simulink model "IEEE30_case"  (R2024b)
settings: Solver=FixedStepAuto  StartTime=0  StopTime=5  FixedStep=1e-7  RelTol=1e-3
values from neighbouring files (symbols this model uses):
  GFL_DFIG_7_C_bus = 0.08    [IEEE30_case_parameters.m]
  GFL_DFIG_7_D_mutual = 2.500000e+3    (= 2500)    [IEEE30_case_parameters.m]
  GFL_DFIG_7_f0 = 60    [IEEE30_case_parameters.m]
  GFL_DFIG_7_gPLLi = 3200    [IEEE30_case_parameters.m]
  GFL_DFIG_7_gPLLp = 650    [IEEE30_case_parameters.m]
  GFL_DFIG_7_H_WT = 0.4    [IEEE30_case_parameters.m]
  GFL_DFIG_7_Hg = 0.8    [IEEE30_case_parameters.m]
  GFL_DFIG_7_Igq_ref = 0    [IEEE30_case_parameters.m]
  GFL_DFIG_7_Ird_ref = 704.45696    [IEEE30_case_parameters.m]
  GFL_DFIG_7_KI_V = -300000    [IEEE30_case_parameters.m]
  GFL_DFIG_7_KP_V = -1000    [IEEE30_case_parameters.m]
  GFL_DFIG_7_Ksh = 1.254300e+4    (= 12543)    [IEEE30_case_parameters.m]
  GFL_DFIG_7_Lg = 0.000483    [IEEE30_case_parameters.m]
  GFL_DFIG_7_Lm_pu = 4    [IEEE30_case_parameters.m]
  GFL_DFIG_7_N = 100    [IEEE30_case_parameters.m]
  GFL_DFIG_7_p = 2    [IEEE30_case_parameters.m]
  GFL_DFIG_7_Pitch = 0    [IEEE30_case_parameters.m]
  GFL_DFIG_7_R = 44    [IEEE30_case_parameters.m]
  GFL_DFIG_7_Rg = 2.000000e-5    (= 2e-05)    [IEEE30_case_parameters.m]
  GFL_DFIG_7_rho = 1.225    [IEEE30_case_parameters.m]
  GFL_DFIG_7_rPLLi = 4500    [IEEE30_case_parameters.m]
  GFL_DFIG_7_rPLLp = 620    [IEEE30_case_parameters.m]
  GFL_DFIG_7_Rs_pu = 0.011    [IEEE30_case_parameters.m]
  GFL_DFIG_7_Sbase = 2.000000e+6    (= 2000000)    [IEEE30_case_parameters.m]
  GFL_DFIG_7_ugq_ref = 0    [IEEE30_case_parameters.m]
  GFL_DFIG_7_usd_ref = 0    [IEEE30_case_parameters.m]
  GFL_DFIG_7_Vbase = 690    [IEEE30_case_parameters.m]
  GFL_DFIG_7_Vdc_ref = 1200    [IEEE30_case_parameters.m]
  GFL_DFIG_7_wind = 12    [IEEE30_case_parameters.m]
  GFL_DFIG_7_wm_ref = 518.184209    [IEEE30_case_parameters.m]
  SG_D_13_D = 0.01056    [IEEE30_case_parameters.m]
  SG_D_13_EnableSaturation = 0    [IEEE30_case_parameters.m]
  SG_D_13_f0 = 60    [IEEE30_case_parameters.m]
  SG_D_13_H = 7.5    [IEEE30_case_parameters.m]
  SG_D_13_K_A = 20    [IEEE30_case_parameters.m]
  SG_D_13_K_E = 1.000000e+1    (= 10)    [IEEE30_case_parameters.m]
  SG_D_13_K_F = 2.363    [IEEE30_case_parameters.m]
  SG_D_13_K_s = 0.5    [IEEE30_case_parameters.m]
  SG_D_13_R_a = 0.001088    [IEEE30_case_parameters.m]
  SG_D_13_S_A = 1    [IEEE30_case_parameters.m]
  SG_D_13_S_B = 0.103    [IEEE30_case_parameters.m]
  SG_D_13_S_N = 10.659857    [IEEE30_case_parameters.m]
  SG_D_13_SpeedPara = 200    [IEEE30_case_parameters.m]
  SG_D_13_T_0 = 0.370163    [IEEE30_case_parameters.m]
  SG_D_13_T_1 = 0.3    [IEEE30_case_parameters.m]
  SG_D_13_T_2 = 0.05    [IEEE30_case_parameters.m]
  SG_D_13_T_3 = 0.02    [IEEE30_case_parameters.m]
  SG_D_13_T_4 = 0.005    [IEEE30_case_parameters.m]
  SG_D_13_T_A = 0.02    [IEEE30_case_parameters.m]
  SG_D_13_T_dd = 8.000000e+0    (= 8)    [IEEE30_case_parameters.m]
  SG_D_13_T_ddd = 0.04    [IEEE30_case_parameters.m]
  SG_D_13_T_E = 0.314    [IEEE30_case_parameters.m]
  SG_D_13_T_F = 0.35    [IEEE30_case_parameters.m]
  SG_D_13_T_qd = 0.8    [IEEE30_case_parameters.m]
  SG_D_13_T_qdd = 0.02    [IEEE30_case_parameters.m]
  SG_D_13_T_speed = 0.1    [IEEE30_case_parameters.m]
  SG_D_13_T_w = 0.5    [IEEE30_case_parameters.m]
  SG_D_13_V_ref = 1.696619    [IEEE30_case_parameters.m]
  SG_D_13_w_ref = 376.991118    [IEEE30_case_parameters.m]
  SG_D_13_x_d = 1.9    [IEEE30_case_parameters.m]
  SG_D_13_x_dd = 0.302    [IEEE30_case_parameters.m]
  SG_D_13_x_ddd = 0.204    [IEEE30_case_parameters.m]
  SG_D_13_x_l = 0.05    [IEEE30_case_parameters.m]
  SG_D_13_x_q = 1.3    [IEEE30_case_parameters.m]
  SG_D_13_x_qd = 0.5    [IEEE30_case_parameters.m]
  SG_D_13_x_qdd = 0.3    [IEEE30_case_parameters.m]
  SG_D_1_D = 0.01056    [IEEE30_case_parameters.m]
  SG_D_1_EnableSaturation = 0    [IEEE30_case_parameters.m]
  SG_D_1_f0 = 60    [IEEE30_case_parameters.m]
  SG_D_1_H = 7.5    [IEEE30_case_parameters.m]
  SG_D_1_K_A = 20    [IEEE30_case_parameters.m]
  SG_D_1_K_E = 1.000000e+1    (= 10)    [IEEE30_case_parameters.m]
  SG_D_1_K_F = 2.363    [IEEE30_case_parameters.m]
  SG_D_1_K_s = 0.5    [IEEE30_case_parameters.m]
  SG_D_1_R_a = 0.001088    [IEEE30_case_parameters.m]
  SG_D_1_S_A = 1    [IEEE30_case_parameters.m]
  SG_D_1_S_B = 0.103    [IEEE30_case_parameters.m]
  SG_D_1_S_N = 10.659857    [IEEE30_case_parameters.m]
  SG_D_1_SpeedPara = 200    [IEEE30_case_parameters.m]
  SG_D_1_T_0 = 0.259812    [IEEE30_case_parameters.m]
  SG_D_1_T_1 = 0.3    [IEEE30_case_parameters.m]
  SG_D_1_T_2 = 0.05    [IEEE30_case_parameters.m]
  SG_D_1_T_3 = 0.02    [IEEE30_case_parameters.m]
  SG_D_1_T_4 = 0.005    [IEEE30_case_parameters.m]
  SG_D_1_T_A = 0.02    [IEEE30_case_parameters.m]
  SG_D_1_T_dd = 8.000000e+0    (= 8)    [IEEE30_case_parameters.m]
  SG_D_1_T_ddd = 0.04    [IEEE30_case_parameters.m]
  SG_D_1_T_E = 0.314    [IEEE30_case_parameters.m]
  SG_D_1_T_F = 0.35    [IEEE30_case_parameters.m]
  SG_D_1_T_qd = 0.8    [IEEE30_case_parameters.m]
  SG_D_1_T_qdd = 0.02    [IEEE30_case_parameters.m]
  SG_D_1_T_speed = 0.1    [IEEE30_case_parameters.m]
  SG_D_1_T_w = 0.5    [IEEE30_case_parameters.m]
  SG_D_1_V_ref = 1.544107    [IEEE30_case_parameters.m]
  SG_D_1_w_ref = 376.991118    [IEEE30_case_parameters.m]
  SG_D_1_x_d = 1.9    [IEEE30_case_parameters.m]
  SG_D_1_x_dd = 0.302    [IEEE30_case_parameters.m]
  SG_D_1_x_ddd = 0.204    [IEEE30_case_parameters.m]
  SG_D_1_x_l = 0.05    [IEEE30_case_parameters.m]
  SG_D_1_x_q = 1.3    [IEEE30_case_parameters.m]
  SG_D_1_x_qd = 0.5    [IEEE30_case_parameters.m]
  SG_D_1_x_qdd = 0.3    [IEEE30_case_parameters.m]
  SG_D_22_D = 0.01056    [IEEE30_case_parameters.m]
  SG_D_22_EnableSaturation = 0    [IEEE30_case_parameters.m]
  SG_D_22_f0 = 60    [IEEE30_case_parameters.m]
  SG_D_22_H = 7.5    [IEEE30_case_parameters.m]
  SG_D_22_K_A = 20    [IEEE30_case_parameters.m]
  SG_D_22_K_E = 1.000000e+1    (= 10)    [IEEE30_case_parameters.m]
  SG_D_22_K_F = 2.363    [IEEE30_case_parameters.m]
  SG_D_22_K_s = 0.5    [IEEE30_case_parameters.m]
  SG_D_22_R_a = 0.001088    [IEEE30_case_parameters.m]
  SG_D_22_S_A = 1    [IEEE30_case_parameters.m]
  SG_D_22_S_B = 0.103    [IEEE30_case_parameters.m]
  SG_D_22_S_N = 10.659857    [IEEE30_case_parameters.m]
  SG_D_22_SpeedPara = 200    [IEEE30_case_parameters.m]
  SG_D_22_T_0 = 0.216121    [IEEE30_case_parameters.m]
  SG_D_22_T_1 = 0.3    [IEEE30_case_parameters.m]
  SG_D_22_T_2 = 0.05    [IEEE30_case_parameters.m]
  SG_D_22_T_3 = 0.02    [IEEE30_case_parameters.m]
  SG_D_22_T_4 = 0.005    [IEEE30_case_parameters.m]
  ... (+126 more)
(part 14 of 27)

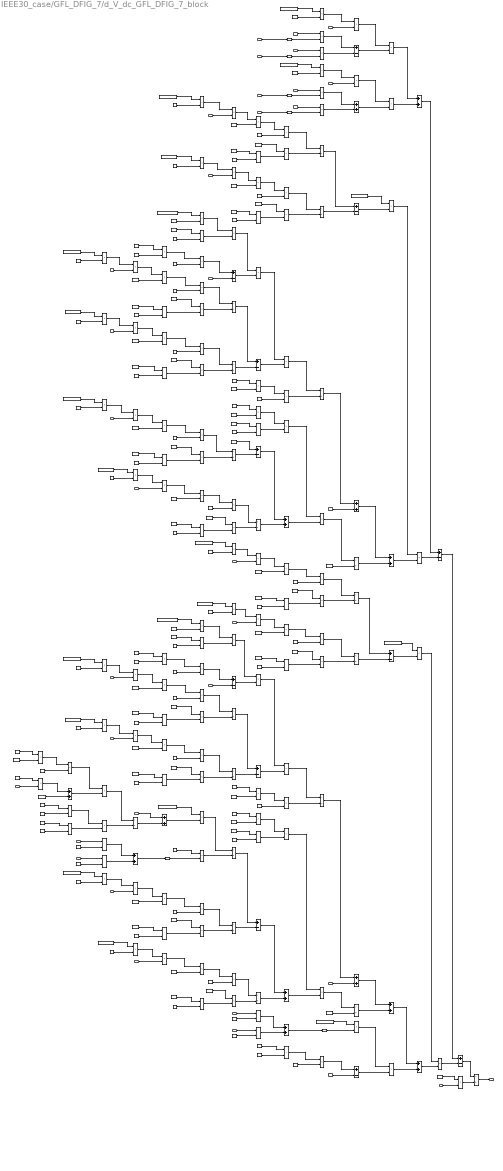
== system IEEE30_case/GFL_DFIG_7/d_V_dc_GFL_DFIG_7_block ==
  note: d_V_dc_GFL_DFIG_7 in IEEE30_case
      | $-\frac{\left(\frac{174.06679757657410473909892168\,\pi \,\Psi _{\mathrm{dr},\mathrm{GFL},\mathrm{DFIG},7}\,\mathrm{Sbase}\,f_{0}}{\mathrm{Lm}_{\mathrm{pu}}\,{\mathrm{Vbase}}^2}-\frac{172.34336393720189526090107832\,\pi \,\Psi _{\mathrm{ds},\mathrm{GFL},\mathrm{DFIG},7}\,\mathrm{Sbase}\,f_{0}}{\mathrm{Lm}_{\mathrm{pu}}\,{\mathrm{Vbase}}^2}\right)\,\left(\Phi _{\mathrm{ra},\mathrm{GFL},\mathrm{DFIG},7}+\frac{1.1\,\mathrm{Rs}_{\mathrm{pu}}\,{\mathrm{Vbase}}^2\,\left(\mathrm{Ird}_{\mathrm{ref}}-\frac{100.497512437811\,\pi \,\Psi _{\mathrm{dr},\mathrm{GFL},\mathrm{DFIG},7}\,\mathrm{Sbase}\,f_{0}}{\mathrm{Lm}_{\mathrm{pu}}\,{\mathrm{Vbase}}^2}+\frac{99.502487562189\,\pi \,\Psi _{\mathrm{ds},\mathrm{GFL},\mathrm{DFIG},7}\,\mathrm{Sbase}\,f_{0}}{\mathrm{Lm}_{\mathrm{pu}}\,{\mathrm{Vbase}}^2}\right)}{\mathrm{Sbase}}+\frac{0.00995049504950496\,\mathrm{Lm}_{\mathrm{pu}}\,{\mathrm{Vbase}}^2\,\left(\frac{100.497512437811\,\pi \,\Psi _{\mathrm{qr},\mathrm{GFL},\mathrm{DFIG},7}\,\mathrm{Sbase}\,f_{0}}{\mathrm{Lm}_{\mathrm{pu}}\,{\mathrm{Vbase}}^2}-\frac{99.502487562189\,\pi \,\Psi _{\mathrm{qs},\mathrm{GFL},\mathrm{DFIG},7}\,\mathrm{Sbase}\,f_{0}}{\mathrm{Lm}_{\mathrm{pu}}\,{\mathrm{Vbase}}^2}\right)\,\left(w_{m,\mathrm{GFL},\mathrm{DFIG},7}-2\,\pi \,f_{0}\right)}{\mathrm{Sbase}\,f_{0}\,\pi }\right)-\left(\frac{174.06679757657410473909892168\,\pi \,\Psi _{\mathrm{qr},\mathrm{GFL},\mathrm{DFIG},7}\,\mathrm{Sbase}\,f_{0}}{\mathrm{Lm}_{\mathrm{pu}}\,{\mathrm{Vbase}}^2}-\frac{172.34336393720189526090107832\,\pi \,\Psi _{\mathrm{qs},\mathrm{GFL},\mathrm{DFIG},7}\,\mathrm{Sbase}\,f_{0}}{\mathrm{Lm}_{\mathrm{pu}}\,{\mathrm{Vbase}}^2}\right)\,\left(0.99009900990099\,\sqrt{{\Psi _{\mathrm{ds},\mathrm{GFL},\mathrm{DFIG},7}}^2+{\Psi _{\mathrm{qs},\mathrm{GFL},\mathrm{DFIG},7}}^2}\,\left(w_{m,\mathrm{GFL},\mathrm{DFIG},7}-2\,\pi \,f_{0}\right)-\Phi _{\mathrm{rb},\mathrm{GFL},\mathrm{DFIG},7}+\frac{1.1\,\mathrm{Rs}_{\mathrm{pu}}\,{\mathrm{Vbase}}^2\,\left(\frac{0.673333333333333\,\Phi _{\mathrm{rc},\mathrm{GFL},\mathrm{DFIG},7}-\frac{10.773333333333328\,\mathrm{Sbase}\,p\,\left(w_{m,\mathrm{GFL},\mathrm{DFIG},7}-\mathrm{wm}_{\mathrm{ref}}\right)}{{f_{0}}^2\,\pi ^2}}{p\,\sqrt{{\Psi _{\mathrm{ds},\mathrm{GFL},\mathrm{DFIG},7}}^2+{\Psi _{\mathrm{qs},\mathrm{GFL},\mathrm{DFIG},7}}^2}}+\frac{100.497512437811\,\pi \,\Psi _{\mathrm{qr},\mathrm{GFL},\mathrm{DFIG},7}\,\mathrm{Sbase}\,f_{0}}{\mathrm{Lm}_{\mathrm{pu}}\,{\mathrm{Vbase}}^2}-\frac{99.502487562189\,\pi \,\Psi _{\mathrm{qs},\mathrm{GFL},\mathrm{DFIG},7}\,\mathrm{Sbase}\,f_{0}}{\mathrm{Lm}_{\mathrm{pu}}\,{\mathrm{Vbase}}^2}\right)}{\mathrm{Sbase}}+\frac{0.00995049504950496\,\mathrm{Lm}_{\mathrm{pu}}\,{\mathrm{Vbase}}^2\,\left(\frac{100.497512437811\,\pi \,\Psi _{\mathrm{dr},\mathrm{GFL},\mathrm{DFIG},7}\,\mathrm{Sbase}\,f_{0}}{\mathrm{Lm}_{\mathrm{pu}}\,{\mathrm{Vbase}}^2}-\frac{99.502487562189\,\pi \,\Psi _{\mathrm{ds},\mathrm{GFL},\mathrm{DFIG},7}\,\mathrm{Sbase}\,f_{0}}{\mathrm{Lm}_{\mathrm{pu}}\,{\mathrm{Vbase}}^2}\right)\,\left(w_{m,\mathrm{GFL},\mathrm{DFIG},7}-2\,\pi \,f_{0}\right)}{\mathrm{Sbase}\,f_{0}\,\pi }\right)+1.73205080756888\,\mathrm{Vbase}\,i_{\mathrm{gd},\mathrm{GFL},\mathrm{DFIG},7}\,\left(v_{d,\mathrm{GFL},\mathrm{DFIG},7}\,\cos\left(\theta _{\mathrm{pllg},\mathrm{GFL},\mathrm{DFIG},7}\right)-v_{q,\mathrm{GFL},\mathrm{DFIG},7}\,\sin\left(\theta _{\mathrm{pllg},\mathrm{GFL},\mathrm{DFIG},7}\right)\right)-1.73205080756888\,\mathrm{Vbase}\,i_{\mathrm{gq},\mathrm{GFL},\mathrm{DFIG},7}\,\left(v_{q,\mathrm{GFL},\mathrm{DFIG},7}\,\cos\left(\theta _{\mathrm{pllg},\mathrm{GFL},\mathrm{DFIG},7}\right)+v_{d,\mathrm{GFL},\mathrm{DFIG},7}\,\sin\left(\theta _{\mathrm{pllg},\mathrm{GFL},\mathrm{DFIG},7}\right)\right)}{C_{\mathrm{bus}}\,V_{\mathrm{dc},\mathrm{GFL},\mathrm{DFIG},7}}$
      | Automatically generated on 2025-11-01 18:33:54 .
  State_i_gd_GFL_DFIG_7_47a9f : Inport
  Input_v_d_GFL_DFIG_7_58356 : Inport  Port=2
  State_theta_pllg_GFL_DFIG_7_c67a2 : Inport  Port=3
  Input_v_q_GFL_DFIG_7_3c611 : Inport  Port=4
  State_theta_pllg_GFL_DFIG_7_35391 : Inport  Port=5
  State_i_gq_GFL_DFIG_7_793b6 : Inport  Port=6
  Input_v_d_GFL_DFIG_7_bbd62 : Inport  Port=7
  State_theta_pllg_GFL_DFIG_7_002e2 : Inport  Port=8
  Input_v_q_GFL_DFIG_7_49107 : Inport  Port=9
  State_theta_pllg_GFL_DFIG_7_66e51 : Inport  Port=10
  State_Psi_dr_GFL_DFIG_7_6e653 : Inport  Port=11
  State_Psi_ds_GFL_DFIG_7_832af : Inport  Port=12
  State_w_m_GFL_DFIG_7_6ca23 : Inport  Port=13
  State_Psi_qr_GFL_DFIG_7_2b0e8 : Inport  Port=14
  State_Psi_qs_GFL_DFIG_7_f70b4 : Inport  Port=15
  State_Phi_ra_GFL_DFIG_7_71e34 : Inport  Port=16
  State_Psi_dr_GFL_DFIG_7_0acea : Inport  Port=17
  State_Psi_ds_GFL_DFIG_7_692c3 : Inport  Port=18
  State_Psi_qr_GFL_DFIG_7_f1f75 : Inport  Port=19
  State_Psi_qs_GFL_DFIG_7_fde33 : Inport  Port=20
  State_w_m_GFL_DFIG_7_73a6c : Inport  Port=21
  State_Psi_dr_GFL_DFIG_7_978cf : Inport  Port=22
  State_Psi_ds_GFL_DFIG_7_2e09c : Inport  Port=23
  State_Phi_rb_GFL_DFIG_7_e2f9d : Inport  Port=24
  State_Phi_rc_GFL_DFIG_7_c7d1c : Inport  Port=25
  State_w_m_GFL_DFIG_7_35e3b : Inport  Port=26
  State_Psi_ds_GFL_DFIG_7_dee5b : Inport  Port=27
  State_Psi_qs_GFL_DFIG_7_f7902 : Inport  Port=28
  State_Psi_qr_GFL_DFIG_7_e69a0 : Inport  Port=29
  State_Psi_qs_GFL_DFIG_7_44146 : Inport  Port=30
  State_Psi_ds_GFL_DFIG_7_a0019 : Inport  Port=31
  State_Psi_qs_GFL_DFIG_7_97bd8 : Inport  Port=32
  State_w_m_GFL_DFIG_7_46811 : Inport  Port=33
  State_V_dc_GFL_DFIG_7_49932 : Inport  Port=34
  Add_18ef7 : Sum
  Add_22a02 : Sum
  Add_4cbdf : Sum
  Add_4f230 : Sum
  Add_5a4e6 : Sum
  Add_9ae8b : Sum
  Add_9b4aa : Sum
  Add_a886b : Sum
  Add_bba29 : Sum
  Add_c2ca7 : Sum
  Add_cdeef : Sum
  Add_d84a0 : Sum
  Add_fa038 : Sum
  Constant_-0.00995049504950496_d1516 : Constant  Value=-0.00995049504950496
  Constant_-0.673333333333333_b8393 : Constant  Value=-0.673333333333333
  Constant_-1.73205080756888_e6adb : Constant  Value=-1.73205080756888
  Constant_-1_13871 : Constant  Value=-1
  Constant_0.00995049504950496_67c00 : Constant  Value=0.00995049504950496
  Constant_0.99009900990099_89273 : Constant  Value=0.99009900990099
  Constant_1.1_36c76 : Constant  Value=1.1
  Constant_1.1_fe12f : Constant  Value=1.1
  Constant_1.73205080756888_198f9 : Constant  Value=1.73205080756888
  Constant_1.73205080756888_62938 : Constant  Value=1.73205080756888
  Constant_1.73205080756888_aa3cb : Constant  Value=1.73205080756888
  Constant_100.497512437811_17d9c : Constant  Value=100.497512437811
  Constant_100.497512437811_19d56 : Constant  Value=100.497512437811
  Constant_100.497512437811_776b8 : Constant  Value=100.497512437811
  Constant_100.497512437811_7e222 : Constant  Value=100.497512437811
  Constant_100.497512437811_d1579 : Constant  Value=100.497512437811
  Constant_100.497512437811_efee0 : Constant  Value=100.497512437811
  Constant_16.0_ca5b8 : Constant  Value=16.0
  Constant_2.0_04737 : Constant  Value=2.0
  Constant_2.0_0e667 : Constant  Value=2.0
  Constant_2.0_147b2 : Constant  Value=2.0
  Constant_2.0_{17682,51112,76025,89488} (4 alike) : Constant  Value=2.0
  Constant_2.0_27d08 : Constant  Value=2.0
  Constant_2.0_28d51 : Constant  Value=2.0
  Constant_2.0_2a2a4 : Constant  Value=2.0
  Constant_2.0_3551f : Constant  Value=2.0
  Constant_2.0_50b33 : Constant  Value=2.0
  Constant_2.0_59ded : Constant  Value=2.0
  Constant_2.0_5dcb4 : Constant  Value=2.0
  Constant_2.0_6f0c1 : Constant  Value=2.0
  Constant_2.0_7f34b : Constant  Value=2.0
  Constant_2.0_8867b : Constant  Value=2.0
  Constant_2.0_9cbdf : Constant  Value=2.0
  Constant_2.0_a00e4 : Constant  Value=2.0
  Constant_2.0_bd6c4 : Constant  Value=2.0
  Constant_2.0_c92ad : Constant  Value=2.0
  Constant_2.0_cbfa6 : Constant  Value=2.0
  Constant_2.0_d2fa3 : Constant  Value=2.0
  Constant_2.0_f082e : Constant  Value=2.0
  Constant_2.0_f4b28 : Constant  Value=2.0
  Constant_99.502487562189_22003 : Constant  Value=99.502487562189
  Constant_99.502487562189_86dbb : Constant  Value=99.502487562189
  Constant_99.502487562189_a4539 : Constant  Value=99.502487562189
  Constant_99.502487562189_b4d1c : Constant  Value=99.502487562189
  Constant_99.502487562189_c6b26 : Constant  Value=99.502487562189
  Constant_99.502487562189_c7b56 : Constant  Value=99.502487562189
  Constant_C_bus_0c2e4 : Constant  Value=C_bus
  Constant_Ird_ref_31f4c : Constant  Value=Ird_ref
  Constant_Lm_pu_09ab7 : Constant  Value=Lm_pu
  Constant_Lm_pu_38274 : Constant  Value=Lm_pu
  Constant_Lm_pu_5aea1 : Constant  Value=Lm_pu
  Constant_Lm_pu_5c3ca : Constant  Value=Lm_pu
  Constant_Lm_pu_63de2 : Constant  Value=Lm_pu
  Constant_Lm_pu_75f63 : Constant  Value=Lm_pu
  Constant_Lm_pu_7d6d9 : Constant  Value=Lm_pu
  Constant_Lm_pu_82642 : Constant  Value=Lm_pu
  Constant_Lm_pu_8d7bc : Constant  Value=Lm_pu
  Constant_Lm_pu_9d1ac : Constant  Value=Lm_pu
  Constant_Lm_pu_a9330 : Constant  Value=Lm_pu
  Constant_Lm_pu_c7022 : Constant  Value=Lm_pu
  Constant_Lm_pu_d357e : Constant  Value=Lm_pu
  Constant_Lm_pu_e166f : Constant  Value=Lm_pu
  Constant_Rs_pu_2c8d3 : Constant  Value=Rs_pu
  Constant_Rs_pu_5185a : Constant  Value=Rs_pu
  Constant_Sbase_00b95 : Constant  Value=Sbase
  Constant_Sbase_02485 : Constant  Value=Sbase
  Constant_Sbase_18cb8 : Constant  Value=Sbase
  Constant_Sbase_2670f : Constant  Value=Sbase
  Constant_Sbase_3cb63 : Constant  Value=Sbase
  Constant_Sbase_4d87a : Constant  Value=Sbase
  Constant_Sbase_5d875 : Constant  Value=Sbase
  Constant_Sbase_64cf6 : Constant  Value=Sbase
  Constant_Sbase_6f1fd : Constant  Value=Sbase
  Constant_Sbase_91220 : Constant  Value=Sbase
  Constant_Sbase_a367d : Constant  Value=Sbase
  Constant_Sbase_b5aae : Constant  Value=Sbase
  Constant_Sbase_da089 : Constant  Value=Sbase
  Constant_Sbase_e4f0a : Constant  Value=Sbase
  Constant_Sbase_f0b29 : Constant  Value=Sbase
  Constant_Sbase_fd0d6 : Constant  Value=Sbase
  Constant_Sbase_ff6a9 : Constant  Value=Sbase
  Constant_Vbase_06283 : Constant  Value=Vbase
  Constant_Vbase_090c3 : Constant  Value=Vbase
  Constant_Vbase_12f2e : Constant  Value=Vbase
  Constant_Vbase_1e3a4 : Constant  Value=Vbase
  Constant_Vbase_227a1 : Constant  Value=Vbase
  Constant_Vbase_2a368 : Constant  Value=Vbase
  Constant_Vbase_2ddd0 : Constant  Value=Vbase
  Constant_Vbase_33a06 : Constant  Value=Vbase
  Constant_Vbase_374be : Constant  Value=Vbase
  Constant_Vbase_5e2df : Constant  Value=Vbase
  Constant_Vbase_80574 : Constant  Value=Vbase
  Constant_Vbase_83da6 : Constant  Value=Vbase
  Constant_Vbase_94783 : Constant  Value=Vbase
  Constant_Vbase_c2293 : Constant  Value=Vbase
  Constant_Vbase_d8c5e : Constant  Value=Vbase
  Constant_Vbase_e9c73 : Constant  Value=Vbase
  Constant_Vbase_f06b6 : Constant  Value=Vbase
  Constant_Vbase_f5330 : Constant  Value=Vbase
  Constant_f0_04506 : Constant  Value=f0
  Constant_f0_07f0c : Constant  Value=f0
  Constant_f0_0d272 : Constant  Value=f0
  Constant_f0_1b018 : Constant  Value=f0
  Constant_f0_35183 : Constant  Value=f0
  Constant_f0_386a1 : Constant  Value=f0
  Constant_f0_39bee : Constant  Value=f0
  Constant_f0_5b664 : Constant  Value=f0
  Constant_f0_7db1c : Constant  Value=f0
  Constant_f0_8327f : Constant  Value=f0
  Constant_f0_856de : Constant  Value=f0
  Constant_f0_978ce : Constant  Value=f0
  Constant_f0_a7e9f : Constant  Value=f0
  Constant_f0_b4361 : Constant  Value=f0
  Constant_f0_bb858 : Constant  Value=f0
  Constant_f0_cbc5f : Constant  Value=f0
  Constant_f0_dad15 : Constant  Value=f0
  Constant_f0_e0a56 : Constant  Value=f0
  Constant_p_26431 : Constant  Value=p
  Constant_p_c592f : Constant  Value=p
  Constant_pi_2370e : Constant  Value=pi
  Constant_pi_2c8c1 : Constant  Value=pi
  Constant_pi_3547f : Constant  Value=pi
  Constant_pi_4281e : Constant  Value=pi
  Constant_pi_42a49 : Constant  Value=pi
  Constant_pi_4a5a6 : Constant  Value=pi
  Constant_pi_66ea4 : Constant  Value=pi
  Constant_pi_69b3f : Constant  Value=pi
  Constant_pi_6a74c : Constant  Value=pi
  Constant_pi_6ca45 : Constant  Value=pi
  Constant_pi_82e36 : Constant  Value=pi
  Constant_pi_a81fe : Constant  Value=pi
  Constant_pi_b655a : Constant  Value=pi
  Constant_pi_c24e4 : Constant  Value=pi
  Constant_pi_c499d : Constant  Value=pi
  Constant_pi_d4cc7 : Constant  Value=pi
  Constant_pi_e36f7 : Constant  Value=pi
  Constant_pi_e9b0b : Constant  Value=pi
  Constant_wm_ref_ae78d : Constant  Value=wm_ref
  Divide_05278 : Product  Inputs=*/
  Divide_0b270 : Product  Inputs=*/
  Divide_183e6 : Product  Inputs=*/
  Divide_2957f : Product  Inputs=*/
  Divide_3375d : Product  Inputs=*/
  Divide_65afe : Product  Inputs=*/
  Divide_69ded : Product  Inputs=*/
  Divide_6d049 : Product  Inputs=*/
  Divide_89f97 : Product  Inputs=*/
  Divide_9053e : Product  Inputs=*/
  Divide_93c9d : Product  Inputs=*/
  Divide_9ef34 : Product  Inputs=*/
  Divide_a2ad4 : Product  Inputs=*/
  Divide_c2c0c : Product  Inputs=*/
  Divide_ce0c1 : Product  Inputs=*/
  Divide_cee0a : Product  Inputs=*/
  Divide_d1818 : Product  Inputs=*/
  Divide_dc6bb : Product  Inputs=*/
  Divide_ec5fc : Product  Inputs=*/
  MathFunc_cos_2cc04 : Trigonometry  Operator=cos
  MathFunc_cos_31ddb : Trigonometry  Operator=cos
  MathFunc_sin_4699a : Trigonometry
  MathFunc_sin_f6f4e : Trigonometry
  MathFunc_sqrt_082b2 : Sqrt
  MathFunc_sqrt_b5fc6 : Sqrt
  Power_04abf : Math  Operator=pow
  Power_{24767,52925,87516,99631} (4 alike) : Math  Operator=pow
  Power_2c4e4 : Math  Operator=pow
  Power_3ba7d : Math  Operator=pow
  Power_40f44 : Math  Operator=pow
  Power_704af : Math  Operator=pow
  Power_791d3 : Math  Operator=pow
  Power_7a399 : Math  Operator=pow
  Power_7be57 : Math  Operator=pow
  Power_83c9c : Math  Operator=pow
  Power_873fd : Math  Operator=pow
  Power_baf20 : Math  Operator=pow
  Power_c24bc : Math  Operator=pow
  Power_c290c : Math  Operator=pow
  Power_c5654 : Math  Operator=pow
  Power_d3eb6 : Math  Operator=pow
  Power_d7c58 : Math  Operator=pow
  Power_e7e7d : Math  Operator=pow
  Power_ed86f : Math  Operator=pow
  Product_0508d : Product
  Product_08651 : Product
  Product_08820 : Product
  Product_0a402 : Product
  Product_0b57f : Product
  Product_0dc02 : Product
  Product_0f050 : Product
  Product_10acf : Product
  Product_15bb3 : Product
  Product_{19635,27306,32718,32795,38056,47171,49245,51009,86797,87140,99528} (11 alike) : Product
  Product_196e6 : Product
  Product_1a315 : Product
  Product_1b517 : Product
  Product_2b3b2 : Product
  Product_2c939 : Product
  Product_2d44b : Product
  Product_2e2b2 : Product
  Product_2ee40 : Product
  Product_33a6f : Product
  Product_394e3 : Product
  Product_3a409 : Product
  Product_3bee8 : Product
  Product_3d7f7 : Product
  Product_3f05c : Product
  Product_44e13 : Product
  Product_4522f : Product
  Product_461c6 : Product
  Product_479e9 : Product
  Product_47cf9 : Product
  Product_47fe3 : Product
  Product_54bf8 : Product
  Product_54eae : Product
  Product_5c6f4 : Product
  Product_5e5d9 : Product
  Product_5ec60 : Product
  Product_5f896 : Product
  Product_61b07 : Product
  Product_6511f : Product
  Product_657aa : Product
  Product_675cd : Product
  Product_6a021 : Product
  Product_6b4f3 : Product
  Product_6eb48 : Product
  Product_6f4ca : Product
  Product_6f5d1 : Product
  Product_6f8bc : Product
  Product_76d01 : Product
  Product_8082a : Product
  Product_817ad : Product
  Product_8e4f6 : Product
  Product_8fb10 : Product
  Product_9253a : Product
  Product_976b9 : Product
  Product_99ee4 : Product
  Product_9a204 : Product
  Product_9e935 : Product
  Product_9f96d : Product
  Product_a1b53 : Product
  Product_a78d3 : Product
  Product_ab4ee : Product
  Product_ac8c8 : Product
  Product_adbf1 : Product
  Product_af0d0 : Product
  Product_af95d : Product
  Product_b28ac : Product
  Product_b3fe9 : Product
  Product_b4507 : Product
  Product_b561e : Product
  Product_b7408 : Product
  Product_bcecc : Product
  Product_bf752 : Product
  Product_bffb9 : Product
  Product_c1fa9 : Product
  Product_c25e0 : Product
  Product_c2a00 : Product
  Product_c2b90 : Product
  Product_c626f : Product
  Product_ca7a8 : Product
  Product_cc40a : Product
  Product_ce605 : Product
  Product_d07be : Product
  Product_d3590 : Product
  Product_d4cc8 : Product
  Product_d704e : Product
  Product_da3fe : Product
  Product_dcec5 : Product
  Product_e0733 : Product
  Product_e0da5 : Product
  Product_e1c1f : Product
  Product_e2792 : Product
  Product_ee904 : Product
  Product_f0431 : Product
  Product_f14b3 : Product
  Product_f308e : Product
  Product_fa6b0 : Product
  Product_fa85b : Product
  Product_fd4c9 : Product
  Product_fefc5 : Product
  Subtract_0e6c0 : Sum  Inputs=+-
  Subtract_44098 : Sum  Inputs=+-
  Subtract_47042 : Sum  Inputs=+-
  Subtract_6a18b : Sum  Inputs=+-
  Subtract_70c7d : Sum  Inputs=+-
  Subtract_7913f : Sum  Inputs=+-
  Subtract_950f7 : Sum  Inputs=+-
  Subtract_ab23c : Sum  Inputs=+-
  Subtract_b4be7 : Sum  Inputs=+-
  Subtract_c350c : Sum  Inputs=+-
  Subtract_c5d86 : Sum  Inputs=+-
  Subtract_f60e6 : Sum  Inputs=+-
  Blockout_d_V_dc_GFL_DFIG_7_1a7e1 : Outport
  wires:
  Add_c2ca7/1 -> Add_9ae8b/1
  Constant_f0_bb858/1 -> Product_ca7a8/2
  State_Psi_dr_GFL_DFIG_7_978cf/1 -> Product_76d01/2
  Product_9a204/1 -> Divide_dc6bb/2
  Constant_Sbase_b5aae/1 -> Product_479e9/2
  Subtract_c5d86/1 -> Divide_93c9d/1
  Power_ed86f/1 -> Add_4cbdf/1
  Constant_Sbase_e4f0a/1 -> Divide_3375d/2
  Product_ce605/1 -> Product_b7408/1
  Divide_93c9d/1 -> Blockout_d_V_dc_GFL_DFIG_7_1a7e1/1
  Product_461c6/1 -> Product_ac8c8/1
  Product_86797/1 -> Divide_3375d/1
  Constant_pi_6ca45/1 -> Product_1a315/2
  Product_bf752/1 -> Divide_93c9d/2
  Constant_Vbase_06283/1 -> Power_7be57/1
  Power_04abf/1 -> Add_4cbdf/2
  Product_d07be/1 -> Product_cc40a/1
  Product_6511f/1 -> Product_b3fe9/1
  Constant_Vbase_090c3/1 -> Power_d3eb6/1
  Product_b28ac/1 -> Product_32718/1
  Constant_Sbase_6f1fd/1 -> Divide_c2c0c/2
  Product_d3590/1 -> Divide_ec5fc/1
  Product_bcecc/1 -> Subtract_c5d86/2
  Product_af95d/1 -> Product_49245/1
  Product_8fb10/1 -> Product_15bb3/1
  Constant_C_bus_0c2e4/1 -> Product_bf752/1
  Product_32795/1 -> Divide_cee0a/1
  State_Psi_qr_GFL_DFIG_7_e69a0/1 -> Product_5e5d9/2
  State_Psi_qs_GFL_DFIG_7_f7902/1 -> Power_704af/1
  Product_9253a/1 -> Product_657aa/1
  Constant_Sbase_3cb63/1 -> Product_fefc5/2
  Subtract_f60e6/1 -> Add_cdeef/1
  Divide_d1818/1 -> Subtract_c350c/1
  Constant_99.502487562189_c7b56/1 -> Product_27306/1
  Constant_0.99009900990099_89273/1 -> Product_b28ac/1
  Product_0a402/1 -> Product_0dc02/1
  Product_3d7f7/1 -> Divide_ec5fc/2
  Constant_pi_c24e4/1 -> Product_461c6/2
  Product_76d01/1 -> Product_a1b53/1
  State_V_dc_GFL_DFIG_7_49932/1 -> Product_bf752/2
  Divide_ec5fc/1 -> Subtract_f60e6/2
  Product_32718/1 -> Add_9ae8b/2
  Constant_pi_b655a/1 -> Product_6f8bc/2
  Divide_05278/1 -> Subtract_b4be7/2
  Add_d84a0/1 -> Add_c2ca7/1
  Constant_Sbase_18cb8/1 -> Product_817ad/2
  Constant_2.0_8867b/1 -> Power_99631/2
  Add_9ae8b/1 -> Product_bcecc/2
  Constant_2.0_bd6c4/1 -> Power_3ba7d/2
  Add_9b4aa/1 -> MathFunc_sqrt_b5fc6/1
  Subtract_70c7d/1 -> Product_08820/2
  Subtract_0e6c0/1 -> Product_32718/2
  Constant_pi_e36f7/1 -> Product_479e9/1
  Product_10acf/1 -> Divide_0b270/1
  Product_ac8c8/1 -> Product_394e3/1
  Divide_3375d/1 -> Add_c2ca7/2
  State_w_m_GFL_DFIG_7_46811/1 -> Subtract_0e6c0/2
  Divide_9ef34/1 -> Subtract_c350c/2
  Product_0dc02/1 -> Divide_65afe/1
  Product_479e9/1 -> Product_08651/1
  Product_ca7a8/1 -> Subtract_0e6c0/1
  Product_6f4ca/1 -> Product_ca7a8/1
  Product_fd4c9/1 -> Product_196e6/1
  Constant_pi_d4cc7/1 -> Product_6f4ca/2
  Product_d4cc8/1 -> Divide_0b270/2
  Constant_f0_07f0c/1 -> Product_c25e0/2
  Constant_2.0_28d51/1 -> Product_6f4ca/1
  MathFunc_cos_2cc04/1 -> Product_6a021/2
  Constant_2.0_04737/1 -> Power_24767/2
  Divide_dc6bb/1 -> Subtract_f60e6/1
  Constant_p_c592f/1 -> Product_a78d3/2
  Add_cdeef/1 -> Product_86797/2
  Constant_Vbase_d8c5e/1 -> Power_99631/1
  Constant_Lm_pu_d357e/1 -> Product_af0d0/1
  Constant_100.497512437811_efee0/1 -> Product_e0733/1
  Constant_2.0_6f0c1/1 -> Power_d7c58/2
  Product_a78d3/1 -> Product_10acf/1
  Constant_Sbase_fd0d6/1 -> Product_a1b53/2
  Product_196e6/1 -> Divide_9ef34/1
  MathFunc_sqrt_082b2/1 -> Product_b28ac/2
  Constant_Lm_pu_8d7bc/1 -> Product_f308e/1
  Divide_9053e/1 -> Subtract_ab23c/2
  Add_4cbdf/1 -> MathFunc_sqrt_082b2/1
  State_Psi_ds_GFL_DFIG_7_a0019/1 -> Power_ed86f/1
  Constant_Sbase_00b95/1 -> Product_394e3/2
  Constant_2.0_59ded/1 -> Power_83c9c/2
  Constant_2.0_51112/1 -> Power_7be57/2
  Product_27306/1 -> Product_675cd/1
  State_Psi_qs_GFL_DFIG_7_44146/1 -> Product_ac8c8/2
  Constant_2.0_9cbdf/1 -> Power_04abf/2
  Product_51009/1 -> Add_bba29/1
  Product_08820/1 -> Divide_a2ad4/1
  State_Psi_qs_GFL_DFIG_7_97bd8/1 -> Power_04abf/1
  State_w_m_GFL_DFIG_7_35e3b/1 -> Product_99528/2
  Product_9f96d/1 -> Product_54bf8/1
  Constant_2.0_c92ad/1 -> Power_ed86f/2
  Power_99631/1 -> Product_f308e/2
  Constant_-0.673333333333333_b8393/1 -> Product_c1fa9/1
  Product_c2a00/1 -> Product_44e13/1
  Product_bffb9/1 -> Product_5e5d9/1
  Product_e2792/1 -> Add_a886b/1
  Divide_ce0c1/1 -> Add_cdeef/2
  Constant_Lm_pu_a9330/1 -> Product_3d7f7/1
  Power_52925/1 -> Product_3f05c/2
  Product_f308e/1 -> Divide_ce0c1/2
  MathFunc_sin_f6f4e/1 -> Product_54eae/2
  Product_c25e0/1 -> Divide_ce0c1/1
  Product_b3fe9/1 -> Product_fd4c9/1
  Constant_100.497512437811_19d56/1 -> Product_bffb9/1
  Constant_f0_856de/1 -> Product_d704e/2
  State_Psi_qr_GFL_DFIG_7_2b0e8/1 -> Product_af95d/2
  Product_6f5d1/1 -> Divide_69ded/2
  Add_4f230/1 -> Product_f0431/2
  Product_394e3/1 -> Product_c25e0/1
  Add_a886b/1 -> Product_6b4f3/2
  Constant_f0_0d272/1 -> Product_08651/2
  Constant_Vbase_12f2e/1 -> Power_7a399/1
  Product_b7408/1 -> Product_3bee8/1
  Constant_Sbase_a367d/1 -> Product_33a6f/2
  Add_fa038/1 -> Product_3bee8/2
  Constant_2.0_17682/1 -> Power_d3eb6/2
  Divide_2957f/1 -> Subtract_b4be7/1
  Constant_99.502487562189_b4d1c/1 -> Product_461c6/1
  Constant_16.0_ca5b8/1 -> Product_fefc5/1
  Product_08651/1 -> Divide_a2ad4/2
  Power_873fd/1 -> Product_4522f/2
  Power_7a399/1 -> Product_3d7f7/2
  State_Psi_qr_GFL_DFIG_7_f1f75/1 -> Product_54bf8/2
  Constant_2.0_f082e/1 -> Power_7a399/2
  Constant_Vbase_33a06/1 -> Product_d07be/2
  Product_dcec5/1 -> Divide_89f97/2
  Constant_f0_8327f/1 -> Product_d3590/2
  Constant_pi_42a49/1 -> Product_bffb9/2
  Product_33a6f/1 -> Product_d3590/1
  Power_baf20/1 -> Product_5ec60/2
  Divide_6d049/1 -> Subtract_70c7d/1
  Product_5e5d9/1 -> Product_33a6f/1
  MathFunc_sqrt_b5fc6/1 -> Product_9a204/2
  State_Psi_qs_GFL_DFIG_7_f70b4/1 -> Product_44e13/2
  Power_704af/1 -> Add_9b4aa/2
  Constant_f0_5b664/1 -> Product_c626f/2
  Constant_2.0_5dcb4/1 -> Power_704af/2
  State_Phi_rc_GFL_DFIG_7_c7d1c/1 -> Add_22a02/1
  Constant_pi_6a74c/1 -> Product_c2a00/2
  Power_e7e7d/1 -> Add_9b4aa/1
  Constant_2.0_3551f/1 -> Power_e7e7d/2
  State_Psi_ds_GFL_DFIG_7_dee5b/1 -> Power_e7e7d/1
  Constant_99.502487562189_a4539/1 -> Product_6511f/1
  Constant_Lm_pu_9d1ac/1 -> Product_47cf9/2
  Constant_p_26431/1 -> Product_9a204/1
  Product_c1fa9/1 -> Divide_dc6bb/1
  Product_2ee40/1 -> Product_da3fe/1
  Add_22a02/1 -> Product_c1fa9/2
  Product_3f05c/1 -> Divide_65afe/2
  Divide_0b270/1 -> Add_22a02/2
  Product_6f8bc/1 -> Product_0508d/1
  Constant_f0_386a1/1 -> Product_0dc02/2
  Constant_Vbase_1e3a4/1 -> Power_3ba7d/1
  Constant_Vbase_94783/1 -> Power_baf20/1
  Constant_Vbase_c2293/1 -> Product_2ee40/2
  Power_c290c/1 -> Product_d4cc8/2
  Constant_0.00995049504950496_67c00/1 -> Product_adbf1/1
  Constant_2.0_50b33/1 -> Power_c290c/2
  Constant_f0_b4361/1 -> Power_c290c/1
  Power_c24bc/1 -> Product_d4cc8/1
  Constant_2.0_147b2/1 -> Power_c24bc/2
  Constant_pi_3547f/1 -> Power_c24bc/1
  Subtract_ab23c/1 -> Product_99ee4/2
  Constant_1.73205080756888_198f9/1 -> Product_6eb48/1
  Add_18ef7/1 -> Product_10acf/2
  Constant_pi_c499d/1 -> Product_9f96d/2
  Constant_pi_4a5a6/1 -> Product_27306/2
  Constant_wm_ref_ae78d/1 -> Add_18ef7/2
  Product_4522f/1 -> Product_fa6b0/1
  State_i_gd_GFL_DFIG_7_47a9f/1 -> Product_cc40a/2
  Constant_Vbase_2a368/1 -> Power_2c4e4/1
  Product_99528/1 -> Add_18ef7/1
  Product_d704e/1 -> Divide_9053e/1
  Constant_-1_13871/1 -> Product_99528/1
  Product_c2b90/1 -> Product_87140/1
  Constant_Lm_pu_7d6d9/1 -> Product_dcec5/1
  Power_40f44/1 -> Product_38056/2
  Product_fefc5/1 -> Product_a78d3/1
  Constant_100.497512437811_776b8/1 -> Product_9f96d/1
  Product_5ec60/1 -> Product_86797/1
  Constant_2.0_76025/1 -> Power_baf20/2
  Product_0508d/1 -> Subtract_47042/1
  Constant_Lm_pu_82642/1 -> Product_8082a/1
  Product_cc40a/1 -> Product_51009/1
  Product_2e2b2/1 -> Product_5ec60/1
  Constant_Rs_pu_2c8d3/1 -> Product_2e2b2/2
  Power_7be57/1 -> Product_3a409/2
  Product_87140/1 -> Product_817ad/1
  Constant_2.0_f4b28/1 -> Power_40f44/2
  Constant_1.1_fe12f/1 -> Product_2e2b2/1
  State_Phi_rb_GFL_DFIG_7_e2f9d/1 -> Add_d84a0/2
  State_Psi_ds_GFL_DFIG_7_692c3/1 -> Product_e1c1f/2
  Divide_69ded/1 -> Add_d84a0/1
  State_Psi_dr_GFL_DFIG_7_6e653/1 -> Product_fa85b/2
  Constant_Ird_ref_31f4c/1 -> Subtract_44098/1
  Constant_f0_35183/1 -> Product_6f5d1/2
  Product_b4507/1 -> Product_6f5d1/1
  Constant_Sbase_4d87a/1 -> Product_b4507/2
  Constant_pi_2370e/1 -> Product_b4507/1
  Constant_2.0_0e667/1 -> Power_873fd/2
  Product_2c939/1 -> Divide_69ded/1
  Subtract_c350c/1 -> Product_2c939/2
  Product_38056/1 -> Divide_9ef34/2
  Product_fa6b0/1 -> Product_08820/1
  Constant_Vbase_227a1/1 -> Power_40f44/1
  Constant_Lm_pu_5c3ca/1 -> Product_38056/1
  Constant_1.73205080756888_62938/1 -> Product_2ee40/1
  Constant_f0_dad15/1 -> Product_196e6/2
  Constant_Sbase_5d875/1 -> Product_fd4c9/2
  State_Psi_ds_GFL_DFIG_7_2e09c/1 -> Product_b3fe9/2
  Product_6a021/1 -> Add_a886b/2
  Product_fa85b/1 -> Product_9253a/1
  Constant_pi_2c8c1/1 -> Product_6511f/2
  Constant_2.0_89488/1 -> Power_87516/2
  Product_e0da5/1 -> Divide_d1818/2
  Power_83c9c/1 -> Product_e0da5/2
  Constant_Vbase_f06b6/1 -> Power_83c9c/1
  Constant_Lm_pu_09ab7/1 -> Product_3a409/1
  Constant_Lm_pu_c7022/1 -> Product_e0da5/1
  Product_2d44b/1 -> Divide_d1818/1
  Product_0f050/1 -> Product_2c939/1
  Constant_f0_978ce/1 -> Product_2d44b/2
  Product_a1b53/1 -> Product_2d44b/1
  Product_675cd/1 -> Product_5c6f4/1
  State_theta_pllg_GFL_DFIG_7_66e51/1 -> MathFunc_cos_2cc04/1
  Product_61b07/1 -> Product_76d01/1
  Product_af0d0/1 -> Divide_183e6/2
  Constant_1.73205080756888_aa3cb/1 -> Product_99ee4/1
  Constant_pi_66ea4/1 -> Product_61b07/2
  Constant_100.497512437811_17d9c/1 -> Product_1a315/1
  Constant_100.497512437811_d1579/1 -> Product_61b07/1
  Product_c626f/1 -> Divide_6d049/1
  Subtract_6a18b/1 -> Product_0f050/2
  State_w_m_GFL_DFIG_7_73a6c/1 -> Subtract_6a18b/2
  Product_15bb3/1 -> Subtract_6a18b/1
  Constant_f0_e0a56/1 -> Product_15bb3/2
  Constant_pi_e9b0b/1 -> Product_8fb10/2
  Constant_2.0_7f34b/1 -> Product_8fb10/1
  Subtract_47042/1 -> Product_fa6b0/2
  Product_8e4f6/1 -> Product_0f050/1
  Power_3ba7d/1 -> Product_8e4f6/2
  Product_adbf1/1 -> Product_8e4f6/1
  State_i_gq_GFL_DFIG_7_793b6/1 -> Product_da3fe/2
  Constant_Lm_pu_75f63/1 -> Product_adbf1/2
  Product_6eb48/1 -> Product_bcecc/1
  Input_v_q_GFL_DFIG_7_49107/1 -> Product_6a021/1
  Subtract_b4be7/1 -> Product_6eb48/2
  Product_8082a/1 -> Divide_05278/2
  Power_2c4e4/1 -> Product_8082a/2
  MathFunc_cos_31ddb/1 -> Product_1b517/2
  Constant_2.0_2a2a4/1 -> Power_2c4e4/2
  Product_9e935/1 -> Divide_05278/1
  Constant_f0_1b018/1 -> Product_9e935/2
  Product_5c6f4/1 -> Product_9e935/1
  Constant_Sbase_da089/1 -> Product_5c6f4/2
  State_Psi_qs_GFL_DFIG_7_fde33/1 -> Product_675cd/2
  Product_47fe3/1 -> Divide_2957f/2
  Power_c5654/1 -> Product_47fe3/2
  Subtract_7913f/1 -> Product_51009/2
  Product_19635/1 -> Product_5f896/1
  Constant_2.0_27d08/1 -> Power_c5654/2
  Constant_Vbase_2ddd0/1 -> Power_c5654/1
  Constant_Lm_pu_e166f/1 -> Product_47fe3/1
  Product_2b3b2/1 -> Divide_2957f/1
  Constant_f0_39bee/1 -> Product_2b3b2/2
  Constant_-1.73205080756888_e6adb/1 -> Product_d07be/1
  Product_ee904/1 -> Product_2b3b2/1
  Constant_Sbase_ff6a9/1 -> Product_ee904/2
  Product_54bf8/1 -> Product_ee904/1
  Subtract_950f7/1 -> Subtract_c5d86/1
  Product_f0431/1 -> Subtract_950f7/2
  Divide_c2c0c/1 -> Add_4f230/2
  Product_3bee8/1 -> Divide_c2c0c/1
  Divide_183e6/1 -> Add_fa038/2
  Power_24767/1 -> Product_af0d0/2
  Constant_Vbase_374be/1 -> Power_24767/1
  Product_47171/1 -> Divide_183e6/1
  Constant_Sbase_f0b29/1 -> Product_0a402/2
  Constant_f0_cbc5f/1 -> Product_47171/2
  Product_0b57f/1 -> Product_47171/1
  Constant_Sbase_91220/1 -> Product_0b57f/2
  Product_e1c1f/1 -> Product_0b57f/1
  Divide_cee0a/1 -> Subtract_44098/2
  Product_da3fe/1 -> Product_6b4f3/1
  Product_b561e/1 -> Product_e1c1f/1
  Constant_pi_69b3f/1 -> Product_b561e/2
  Constant_99.502487562189_86dbb/1 -> Product_b561e/1
  Product_49245/1 -> Product_c626f/1
  Subtract_44098/1 -> Add_fa038/1
  Product_ab4ee/1 -> Divide_cee0a/2
  Power_791d3/1 -> Product_ab4ee/2
  Power_87516/1 -> Product_976b9/2
  Constant_2.0_a00e4/1 -> Power_791d3/2
  MathFunc_sin_4699a/1 -> Product_e2792/2
  Constant_Vbase_80574/1 -> Power_791d3/1
  Constant_Lm_pu_63de2/1 -> Product_ab4ee/1
  Constant_f0_a7e9f/1 -> Product_32795/2
  Product_817ad/1 -> Product_32795/1
  State_Psi_dr_GFL_DFIG_7_0acea/1 -> Product_87140/2
  Constant_pi_82e36/1 -> Product_c2b90/2
  Constant_2.0_cbfa6/1 -> Product_6f8bc/1
  Constant_100.497512437811_7e222/1 -> Product_c2b90/1
  Power_d7c58/1 -> Product_b7408/2
  Constant_Vbase_f5330/1 -> Power_d7c58/1
  Constant_Rs_pu_5185a/1 -> Product_ce605/2
  Constant_1.1_36c76/1 -> Product_ce605/1
  Add_5a4e6/1 -> Add_4f230/1
  Input_v_q_GFL_DFIG_7_3c611/1 -> Product_54eae/1
  State_Phi_ra_GFL_DFIG_7_71e34/1 -> Add_5a4e6/2
  Divide_a2ad4/1 -> Add_5a4e6/1
  Input_v_d_GFL_DFIG_7_58356/1 -> Product_1b517/1
  Product_99ee4/1 -> Product_f0431/1
  Constant_Sbase_02485/1 -> Product_5f896/2
  Divide_65afe/1 -> Subtract_70c7d/2
  Constant_2.0_d2fa3/1 -> Power_52925/2
  Add_bba29/1 -> Subtract_950f7/1
  Constant_Vbase_83da6/1 -> Power_52925/1
  Constant_Lm_pu_5aea1/1 -> Product_3f05c/1
  Product_44e13/1 -> Product_0a402/1
  Constant_99.502487562189_22003/1 -> Product_c2a00/1
  Product_976b9/1 -> Divide_6d049/2
  Constant_Vbase_5e2df/1 -> Power_87516/1
  Constant_Lm_pu_38274/1 -> Product_976b9/1
  Constant_pi_a81fe/1 -> Product_f14b3/2
  Constant_Sbase_2670f/1 -> Product_49245/2
  Product_e0733/1 -> Product_af95d/1
  Constant_pi_4281e/1 -> Product_e0733/2
  State_w_m_GFL_DFIG_7_6ca23/1 -> Subtract_47042/2
  Constant_f0_7db1c/1 -> Product_0508d/2
  Divide_89f97/1 -> Subtract_ab23c/1
  Constant_Vbase_e9c73/1 -> Power_873fd/1
  Product_47cf9/1 -> Product_4522f/1
  Constant_-0.00995049504950496_d1516/1 -> Product_47cf9/1
  Product_3a409/1 -> Divide_9053e/2
  Product_5f896/1 -> Product_d704e/1
  State_Psi_ds_GFL_DFIG_7_832af/1 -> Product_19635/2
  Product_f14b3/1 -> Product_19635/1
  Constant_99.502487562189_c6b26/1 -> Product_f14b3/1
  Power_d3eb6/1 -> Product_dcec5/2
  Product_657aa/1 -> Divide_89f97/1
  Constant_f0_04506/1 -> Product_657aa/2
  Constant_Sbase_64cf6/1 -> Product_9253a/2
  Product_1a315/1 -> Product_fa85b/1
  Product_54eae/1 -> Subtract_7913f/2
  Product_6b4f3/1 -> Add_bba29/2
  Product_1b517/1 -> Subtract_7913f/1
  State_theta_pllg_GFL_DFIG_7_002e2/1 -> MathFunc_sin_4699a/1
  Input_v_d_GFL_DFIG_7_bbd62/1 -> Product_e2792/1
  State_theta_pllg_GFL_DFIG_7_35391/1 -> MathFunc_sin_f6f4e/1
  State_theta_pllg_GFL_DFIG_7_c67a2/1 -> MathFunc_cos_31ddb/1

== system IEEE30_case/GFL_DFIG_7/d_i_gd_GFL_DFIG_7_block ==
  note: d_i_gd_GFL_DFIG_7 in IEEE30_case
      | $\frac{\Phi _{\mathrm{gb},\mathrm{GFL},\mathrm{DFIG},7}-\mathrm{Rg}\,i_{\mathrm{gd},\mathrm{GFL},\mathrm{DFIG},7}+\left(\mathrm{Rg}-4\,\pi \,\mathrm{Lg}\,f_{0}\right)\,\left(i_{\mathrm{gd},\mathrm{GFL},\mathrm{DFIG},7}-\frac{0.666666666666667\,\Phi _{\mathrm{gc},\mathrm{GFL},\mathrm{DFIG},7}-0.666666666666667\,\mathrm{KP}_{V}\,\left(V_{\mathrm{dc},\mathrm{GFL},\mathrm{DFIG},7}-\mathrm{Vdc}_{\mathrm{ref}}\right)}{\mathrm{Vbase}}\right)}{\mathrm{Lg}}$
      | Automatically generated on 2025-11-01 18:33:59 .
  State_Phi_gb_GFL_DFIG_7_1acd8 : Inport
  State_i_gd_GFL_DFIG_7_e096c : Inport  Port=2
  State_i_gd_GFL_DFIG_7_79282 : Inport  Port=3
  State_V_dc_GFL_DFIG_7_27989 : Inport  Port=4
  State_Phi_gc_GFL_DFIG_7_ffb8d : Inport  Port=5
  Add_1ca69 : Sum
  Add_2ed53 : Sum
  Add_571e5 : Sum
  Add_65f35 : Sum
  Constant_-1_343bc : Constant  Value=-1
  Constant_-1_586ef : Constant  Value=-1
  Constant_0.666666666666667_ecfb7 : Constant  Value=0.666666666666667
  Constant_4.0_dfc1f : Constant  Value=4.0
  Constant_KP_V_06cbe : Constant  Value=KP_V
  Constant_Lg_522ee : Constant  Value=Lg
  Constant_Lg_eb38c : Constant  Value=Lg
  Constant_Rg_591a4 : Constant  Value=Rg
  Constant_Rg_dd510 : Constant  Value=Rg
  Constant_Vbase_21c10 : Constant  Value=Vbase
  Constant_Vdc_ref_0a7b6 : Constant  Value=Vdc_ref
  Constant_f0_b76dd : Constant  Value=f0
  Constant_pi_4bccd : Constant  Value=pi
  Divide_21e2e : Product  Inputs=*/
  Divide_6a006 : Product  Inputs=*/
  Product_415af : Product
  Product_5b248 : Product
  Product_66e8e : Product
  Product_67a5a : Product
  Product_a3c71 : Product
  Product_c5a6e : Product
  Product_e6068 : Product
  Product_e65ff : Product
  Product_ebbdb : Product
  Subtract_8389b : Sum  Inputs=+-
  Subtract_a0357 : Sum  Inputs=+-
  Blockout_d_i_gd_GFL_DFIG_7_cd2cb : Outport
  wires:
  Constant_-1_343bc/1 -> Product_66e8e/1
  Product_ebbdb/1 -> Subtract_8389b/2
  State_Phi_gc_GFL_DFIG_7_ffb8d/1 -> Add_571e5/2
  State_i_gd_GFL_DFIG_7_e096c/1 -> Product_ebbdb/2
  State_V_dc_GFL_DFIG_7_27989/1 -> Product_66e8e/2
  Product_66e8e/1 -> Add_2ed53/1
  Constant_Vdc_ref_0a7b6/1 -> Add_2ed53/2
  Add_2ed53/1 -> Product_a3c71/2
  Constant_KP_V_06cbe/1 -> Product_a3c71/1
  Product_a3c71/1 -> Add_571e5/1
  Constant_4.0_dfc1f/1 -> Product_e6068/1
  Constant_pi_4bccd/1 -> Product_e6068/2
  Constant_0.666666666666667_ecfb7/1 -> Product_5b248/1
  Add_571e5/1 -> Product_5b248/2
  Constant_f0_b76dd/1 -> Product_c5a6e/2
  Constant_-1_586ef/1 -> Product_415af/1
  Product_e6068/1 -> Product_67a5a/1
  Constant_Lg_eb38c/1 -> Product_67a5a/2
  State_i_gd_GFL_DFIG_7_79282/1 -> Product_415af/2
  Product_5b248/1 -> Divide_6a006/1
  Constant_Vbase_21c10/1 -> Divide_6a006/2
  Product_67a5a/1 -> Product_c5a6e/1
  Constant_Rg_591a4/1 -> Product_ebbdb/1
  Subtract_8389b/1 -> Add_65f35/1
  Product_415af/1 -> Add_1ca69/1
  Divide_6a006/1 -> Add_1ca69/2
  Product_c5a6e/1 -> Subtract_a0357/1
  Add_65f35/1 -> Divide_21e2e/1
  Constant_Rg_dd510/1 -> Subtract_a0357/2
  State_Phi_gb_GFL_DFIG_7_1acd8/1 -> Subtract_8389b/1
  Add_1ca69/1 -> Product_e65ff/1
  Subtract_a0357/1 -> Product_e65ff/2
  Product_e65ff/1 -> Add_65f35/2
  Constant_Lg_522ee/1 -> Divide_21e2e/2
  Divide_21e2e/1 -> Blockout_d_i_gd_GFL_DFIG_7_cd2cb/1

== system IEEE30_case/GFL_DFIG_7/d_i_gq_GFL_DFIG_7_block ==
  note: d_i_gq_GFL_DFIG_7 in IEEE30_case
      | $-\frac{\mathrm{Rg}\,i_{\mathrm{gq},\mathrm{GFL},\mathrm{DFIG},7}-\Phi _{\mathrm{ga},\mathrm{GFL},\mathrm{DFIG},7}+\left(\mathrm{Rg}-4\,\pi \,\mathrm{Lg}\,f_{0}\right)\,\left(\mathrm{Igq}_{\mathrm{ref}}-i_{\mathrm{gq},\mathrm{GFL},\mathrm{DFIG},7}\right)}{\mathrm{Lg}}$
      | Automatically generated on 2025-11-01 18:34:01 .
  State_Phi_ga_GFL_DFIG_7_1abf4 : Inport
  State_i_gq_GFL_DFIG_7_3f6ab : Inport  Port=2
  State_i_gq_GFL_DFIG_7_5be6d : Inport  Port=3
  Add_1289c : Sum
  Constant_4.0_26018 : Constant  Value=4.0
  Constant_Igq_ref_acf97 : Constant  Value=Igq_ref
  Constant_Lg_928ef : Constant  Value=Lg
  Constant_Lg_99dcb : Constant  Value=Lg
  Constant_Rg_60a4a : Constant  Value=Rg
  Constant_Rg_ebb5a : Constant  Value=Rg
  Constant_f0_bb068 : Constant  Value=f0
  Constant_pi_369a0 : Constant  Value=pi
  Divide_1a938 : Product  Inputs=*/
  Product_4c524 : Product
  Product_59448 : Product
  Product_9f8bc : Product
  Product_cc55a : Product
  Product_dea2c : Product
  Subtract_5876d : Sum  Inputs=+-
  Subtract_68ca5 : Sum  Inputs=+-
  Subtract_794e0 : Sum  Inputs=+-
  Blockout_d_i_gq_GFL_DFIG_7_79c3a : Outport
  wires:
  Constant_pi_369a0/1 -> Product_59448/2
  Constant_4.0_26018/1 -> Product_59448/1
  Product_59448/1 -> Product_dea2c/1
  Constant_Lg_928ef/1 -> Product_dea2c/2
  Product_dea2c/1 -> Product_cc55a/1
  Constant_f0_bb068/1 -> Product_cc55a/2
  Constant_Rg_60a4a/1 -> Product_9f8bc/1
  State_i_gq_GFL_DFIG_7_3f6ab/1 -> Product_9f8bc/2
  Constant_Igq_ref_acf97/1 -> Subtract_68ca5/1
  State_i_gq_GFL_DFIG_7_5be6d/1 -> Subtract_68ca5/2
  Product_cc55a/1 -> Subtract_794e0/1
  Constant_Rg_ebb5a/1 -> Subtract_794e0/2
  State_Phi_ga_GFL_DFIG_7_1abf4/1 -> Subtract_5876d/1
  Product_9f8bc/1 -> Subtract_5876d/2
  Subtract_68ca5/1 -> Product_4c524/1
  Subtract_794e0/1 -> Product_4c524/2
  Subtract_5876d/1 -> Add_1289c/1
  Product_4c524/1 -> Add_1289c/2
  Add_1289c/1 -> Divide_1a938/1
  Constant_Lg_99dcb/1 -> Divide_1a938/2
  Divide_1a938/1 -> Blockout_d_i_gq_GFL_DFIG_7_79c3a/1

== system IEEE30_case/GFL_DFIG_7/d_shaft_w_GFL_DFIG_7_block ==
  note: d_shaft_w_GFL_DFIG_7 in IEEE30_case
      | $\mathrm{Turbine}_{w,\mathrm{GFL},\mathrm{DFIG},7}-\frac{w_{m,\mathrm{GFL},\mathrm{DFIG},7}}{p}$
      | Automatically generated on 2025-11-01 18:33:08 .
  State_Turbine_w_GFL_DFIG_7_fd30f : Inport
  State_w_m_GFL_DFIG_7_93de0 : Inport  Port=2
  Constant_p_7c272 : Constant  Value=p
  Divide_e7f48 : Product  Inputs=*/
  Subtract_9bc0a : Sum  Inputs=+-
  Blockout_d_shaft_w_GFL_DFIG_7_0b709 : Outport
  wires:
  State_Turbine_w_GFL_DFIG_7_fd30f/1 -> Subtract_9bc0a/1
  State_w_m_GFL_DFIG_7_93de0/1 -> Divide_e7f48/1
  Constant_p_7c272/1 -> Divide_e7f48/2
  Divide_e7f48/1 -> Subtract_9bc0a/2
  Subtract_9bc0a/1 -> Blockout_d_shaft_w_GFL_DFIG_7_0b709/1

== system IEEE30_case/GFL_DFIG_7/d_theta_pllg_GFL_DFIG_7_block ==
  note: d_theta_pllg_GFL_DFIG_7 in IEEE30_case
      | $\mathrm{Phipllg}_{\mathrm{GFL},\mathrm{DFIG},7}-\mathrm{gPLLp}\,\left(\mathrm{ugq}_{\mathrm{ref}}+v_{q,\mathrm{GFL},\mathrm{DFIG},7}\,\cos\left(\theta _{\mathrm{pllg},\mathrm{GFL},\mathrm{DFIG},7}\right)+v_{d,\mathrm{GFL},\mathrm{DFIG},7}\,\sin\left(\theta _{\mathrm{pllg},\mathrm{GFL},\mathrm{DFIG},7}\right)\right)$
      | Automatically generated on 2025-11-01 18:34:10 .
  State_Phipllg_GFL_DFIG_7_ae55c : Inport
  Input_v_d_GFL_DFIG_7_973c5 : Inport  Port=2
  State_theta_pllg_GFL_DFIG_7_2f4db : Inport  Port=3
  Input_v_q_GFL_DFIG_7_c7c1e : Inport  Port=4
  State_theta_pllg_GFL_DFIG_7_b3c0b : Inport  Port=5
  Add_0897b : Sum
  Constant_-1_26b2d : Constant  Value=-1
  Constant_gPLLp_235a6 : Constant  Value=gPLLp
  Constant_ugq_ref_9f78d : Constant  Value=ugq_ref
  MathFunc_cos_8cc42 : Trigonometry  Operator=cos
  MathFunc_sin_31c04 : Trigonometry
  Product_05a43 : Product
  Product_56ce4 : Product
  Product_58fcb : Product
  Product_6784f : Product
  Subtract_17aae : Sum  Inputs=+-
  Subtract_9bd15 : Sum  Inputs=+-
  Blockout_d_theta_pllg_GFL_DFIG_7_9b0fc : Outport
  wires:
  State_theta_pllg_GFL_DFIG_7_2f4db/1 -> MathFunc_sin_31c04/1
  MathFunc_sin_31c04/1 -> Product_58fcb/2
  Constant_-1_26b2d/1 -> Product_56ce4/1
  Input_v_d_GFL_DFIG_7_973c5/1 -> Product_58fcb/1
  Constant_ugq_ref_9f78d/1 -> Product_56ce4/2
  State_theta_pllg_GFL_DFIG_7_b3c0b/1 -> MathFunc_cos_8cc42/1
  Product_56ce4/1 -> Subtract_17aae/1
  Product_58fcb/1 -> Subtract_17aae/2
  Input_v_q_GFL_DFIG_7_c7c1e/1 -> Product_6784f/1
  MathFunc_cos_8cc42/1 -> Product_6784f/2
  Subtract_17aae/1 -> Subtract_9bd15/1
  Product_6784f/1 -> Subtract_9bd15/2
  Constant_gPLLp_235a6/1 -> Product_05a43/1
  Subtract_9bd15/1 -> Product_05a43/2
  Add_0897b/1 -> Blockout_d_theta_pllg_GFL_DFIG_7_9b0fc/1
  State_Phipllg_GFL_DFIG_7_ae55c/1 -> Add_0897b/1
  Product_05a43/1 -> Add_0897b/2

== system IEEE30_case/GFL_DFIG_7/d_theta_pllr_GFL_DFIG_7_block ==
  note: d_theta_pllr_GFL_DFIG_7 in IEEE30_case
      | $\mathrm{Phipllr}_{\mathrm{GFL},\mathrm{DFIG},7}-\mathrm{rPLLp}\,\left(\mathrm{usd}_{\mathrm{ref}}+v_{d,\mathrm{GFL},\mathrm{DFIG},7}\,\cos\left(\theta _{\mathrm{pllr},\mathrm{GFL},\mathrm{DFIG},7}\right)-v_{q,\mathrm{GFL},\mathrm{DFIG},7}\,\sin\left(\theta _{\mathrm{pllr},\mathrm{GFL},\mathrm{DFIG},7}\right)\right)$
      | Automatically generated on 2025-11-01 18:34:07 .
  State_Phipllr_GFL_DFIG_7_8b535 : Inport
  Input_v_d_GFL_DFIG_7_57b0c : Inport  Port=2
  State_theta_pllr_GFL_DFIG_7_64a08 : Inport  Port=3
  Input_v_q_GFL_DFIG_7_cdd0f : Inport  Port=4
  State_theta_pllr_GFL_DFIG_7_76fa6 : Inport  Port=5
  Add_79054 : Sum
  Add_88ae6 : Sum
  Constant_-1_3cc9b : Constant  Value=-1
  Constant_rPLLp_323b9 : Constant  Value=rPLLp
  Constant_usd_ref_8ae3d : Constant  Value=usd_ref
  MathFunc_cos_5e566 : Trigonometry  Operator=cos
  MathFunc_sin_c0ea2 : Trigonometry
  Product_73d92 : Product
  Product_7d317 : Product
  Product_845a2 : Product
  Product_f1281 : Product
  Subtract_501fa : Sum  Inputs=+-
  Blockout_d_theta_pllr_GFL_DFIG_7_2facc : Outport
  wires:
  State_theta_pllr_GFL_DFIG_7_64a08/1 -> MathFunc_cos_5e566/1
  Add_79054/1 -> Blockout_d_theta_pllr_GFL_DFIG_7_2facc/1
  MathFunc_cos_5e566/1 -> Product_73d92/2
  Constant_-1_3cc9b/1 -> Product_7d317/1
  Constant_usd_ref_8ae3d/1 -> Product_7d317/2
  Input_v_d_GFL_DFIG_7_57b0c/1 -> Product_73d92/1
  State_theta_pllr_GFL_DFIG_7_76fa6/1 -> MathFunc_sin_c0ea2/1
  Product_7d317/1 -> Subtract_501fa/1
  Product_73d92/1 -> Subtract_501fa/2
  Input_v_q_GFL_DFIG_7_cdd0f/1 -> Product_f1281/1
  MathFunc_sin_c0ea2/1 -> Product_f1281/2
  Subtract_501fa/1 -> Add_88ae6/1
  Product_f1281/1 -> Add_88ae6/2
  Constant_rPLLp_323b9/1 -> Product_845a2/1
  Add_88ae6/1 -> Product_845a2/2
  State_Phipllr_GFL_DFIG_7_8b535/1 -> Add_79054/1
  Product_845a2/1 -> Add_79054/2
